simulink model "General_2_2025a"  (R2025a)
settings: Solver=ode45  StartTime=0.0  StopTime=inf  FixedStep=.1  RelTol=1e-3
undefined symbols (not defined in the file or in its folder): CR, dspblkCoreblockFVToolHelper, gcbh, LF, R_vec
libraries: instrumentseriallib x3, slpidlib x1, simulink x1
settings Model: Creator=aceve  LastModifiedBy=diego

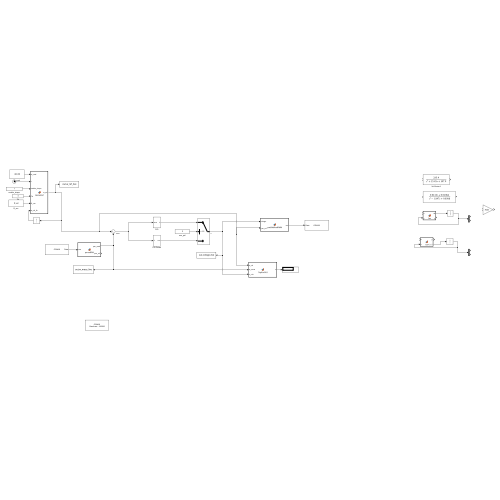
[thumbnail: Simulink's stored preview of the top-level diagram]
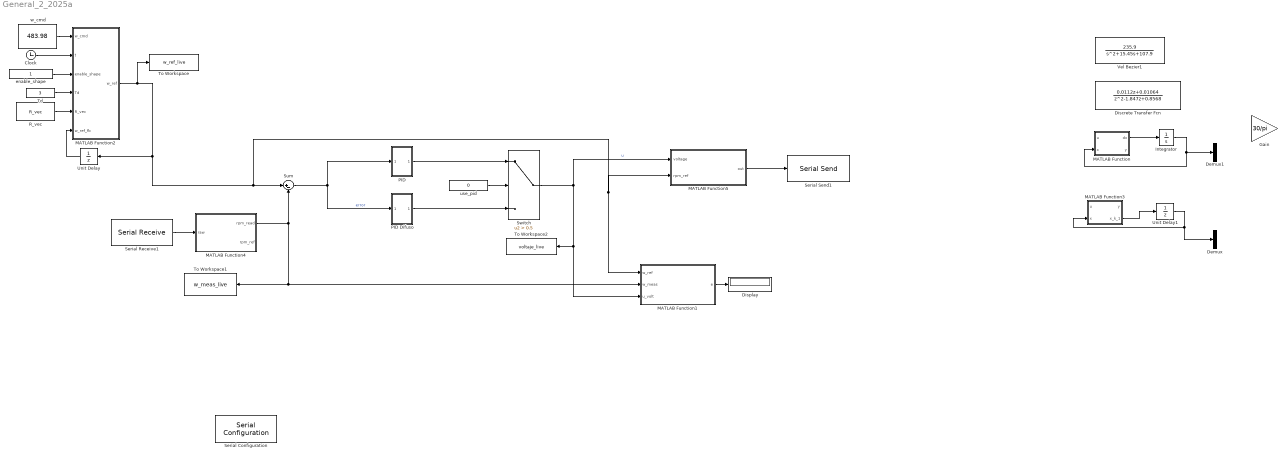
== system General_2_2025a ==
  Clock : Clock
  Demux : Demux  Outputs=2
  Demux1 : Demux  Outputs=2
  Discrete Transfer Fcn : DiscreteTransferFcn  LoadFcn=dspblkCoreblockFVToolHelper(gcbh,'load');  Numerator=[0.0112 0.01064 ]  Denominator=[1 -1.847 0.8568]
      settings: CopyFcn=dspblkCoreblockFVToolHelper(gcbh,'copy');  DeleteFcn=dspblkCoreblockFVToolHelper(gcbh,'close');  ModelCloseFcn=dspblkCoreblockFVToolHelper(gcbh,'close');  PreSaveFcn=dspblkCoreblockFVToolHelper(gcbh,'presave');  PostSaveFcn=dspblkCoreblockFVToolHelper(gcbh,'postsave');  CloseFcn=dspblkCoreblockFVToolHelper(gcbh,'close');
  Display : Display
  Gain : Gain  Gain=30/pi
  Integrator : Integrator  InitialCondition=[0;0]
  MATLAB Function : MATLAB Function  TreatAsAtomicUnit=on
  MATLAB Function1 : MATLAB Function  TreatAsAtomicUnit=on
  MATLAB Function2 : MATLAB Function  TreatAsAtomicUnit=on
  MATLAB Function3 : MATLAB Function  TreatAsAtomicUnit=on
  MATLAB Function4 : MATLAB Function  TreatAsAtomicUnit=on
  MATLAB Function5 : MATLAB Function  TreatAsAtomicUnit=on
  PID : Subsystem
  PID Difuso : Subsystem
  R_vec : Constant  Value=R_vec  SampleTime=-1
  Serial Configuration : instrumentseriallib/Serial Configuration  Priority=-200000  PortSel=COM19  Port=COM19  ComPort=COM19  BaudRate=115200  DataBits=8  Parity=none  StopBits=1  ByteOrder=little-endian  FlowControl=none  Timeout=10  SimulateUsing=Interpreted execution  BlockInModel=on  aMode=1
  Serial Receive1 : instrumentseriallib/Serial Receive  Priority=1  PortSel=COM19  Port=COM19  ComPort=COM19  DataType=int16  SaveDataType=uint8  ToggleHeader=off  Header=[]  ToggleDataSize=on  DataSize=[2 1]  ToggleTerminator=off  Terminator=CR/LF ('\r\n')  CustomTerminator=[]  InputFormat=Column major  EnableBlockingMode=on  ActionDataUnavailable=Output last received value  ActionWhenDataUnavailable=Output last received value  CustomValue=0  SampleTime=0.01  SimulateUsing=Interpreted execution  BlockInModel=on  aMode=1  LibraryInUse=instrumentlib
  Serial Send1 : instrumentseriallib/Serial Send  Priority=1  PortSel=COM19  Port=COM19  ComPort=COM19  Header=[]  Terminator=<none>  CustomTerminator=[]  EnableBlockingMode=off  SimulateUsing=Interpreted execution  BlockInModel=on  aMode=1
  Sum : Sum  Inputs=|+-
  Switch : Switch  Criteria=u2 > Threshold  Threshold=0.5  SaturateOnIntegerOverflow=off  InputSameDT=off
  Td : Constant  Value=3  SampleTime=-1
  To Workspace : ToWorkspace  VariableName=w_ref_live  SampleTime=-1
      settings: MaxDataPoints=1
  To Workspace1 : ToWorkspace  VariableName=w_meas_live  SampleTime=-1
      settings: MaxDataPoints=1
  To Workspace2 : ToWorkspace  VariableName=voltaje_live  SampleTime=-1
      settings: MaxDataPoints=1
  Unit Delay : UnitDelay  SampleTime=-1  HasFrameUpgradeWarning=on
  Unit Delay1 : UnitDelay  InitialCondition=[0;0]  SampleTime=-1  HasFrameUpgradeWarning=on
  Vel Bezier1 : TransferFcn  Numerator=[235.9]  Denominator=[1 15.45 107.9]
  enable_shape : Constant  SampleTime=-1
  use_pid : Constant  Value=0  SampleTime=-1
  w_cmd : Constant  Value=483.98  SampleTime=-1
  wires:
  PID/1(Out1) -> Switch/1
  use_pid/1 -> Switch/2
  Sum/1 -> PID/1(error), PID Difuso/1(In1)  "error"
  MATLAB Function2/1(w_ref) -> Sum/1, MATLAB Function1/1(w_ref), MATLAB Function5/2(rpm_ref), Unit Delay/1, To Workspace/1
  MATLAB Function1/1(e) -> Display/1
  R_vec/1 -> MATLAB Function2/5(R_vec)
  Clock/1 -> MATLAB Function2/2(t)
  Td/1 -> MATLAB Function2/4(Td)
  Unit Delay/1 -> MATLAB Function2/6(w_ref_fb)
  w_cmd/1 -> MATLAB Function2/1(w_cmd)
  enable_shape/1 -> MATLAB Function2/3(enable_shape)
  PID Difuso/1(out) -> Switch/3
  Switch/1 -> MATLAB Function1/3(u_volt), To Workspace2/1, MATLAB Function5/1(voltage)  "u"
  Integrator/1 -> Demux1/1, MATLAB Function/2(x)
  MATLAB Function/1(dx) -> Integrator/1
  MATLAB Function3/2(x_k_1) -> Unit Delay1/1
  Unit Delay1/1 -> Demux/1, MATLAB Function3/2(x)
  Serial Receive1/1 -> MATLAB Function4/1(raw)
  MATLAB Function5/1(out) -> Serial Send1/1
  MATLAB Function4/1(rpm_read) -> MATLAB Function1/2(w_meas), To Workspace1/1, Sum/2

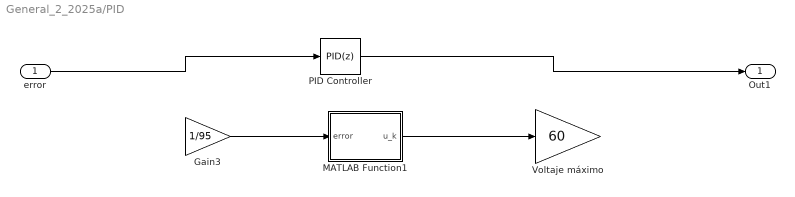
== system General_2_2025a/PID ==
  error : Inport
  Gain3 : Gain  Gain=1/95
  MATLAB Function1 : MATLAB Function  TreatAsAtomicUnit=on
  PID Controller : slpidlib/PID Controller  Controller=PID  Form=Parallel  TimeDomain=Discrete-time  UseExternalTs=off  SampleTime=0.01  IntegratorMethod=Forward Euler  FilterMethod=Forward Euler  ControllerParametersSource=internal  P=1.4156  I=177.0763  UseKiTs=off  D=0.038567  UseExternalDerivativeSource=off  N=9968.78766  UseFilter=on  TunerSelectOption=Transfer Function Based (PID Tuner App)  InitialConditionSource=internal  InitialConditionForIntegrator=0  InitialConditionForFilter=0  DifferentiatorICPrevScaledInput=0  ExternalReset=none  TrackingMode=off  Kt=1  LimitOutput=off  SatLimitsSource=internal  UpperSaturationLimit=inf  LowerSaturationLimit=-inf  LinearizeAsGain=on  AntiWindupMode=none  Kb=1  LimitIntegrator=off  UpperIntegratorSaturationLimit=inf  LowerIntegratorSaturationLimit=-inf  POutMin=[]  POutMax=[]  IOutMin=[]  IOutMax=[]  DOutMin=[]  DOutMax=[]  NOutMin=[]  NOutMax=[]  SumOutMin=[]  SumOutMax=[]  SaturationOutMin=[]  SaturationOutMax=[]  PParamMin=[]  PParamMax=[]  IParamMin=[]  IParamMax=[]  DParamMin=[]  DParamMax=[]  NParamMin=[]  NParamMax=[]  KbParamMin=[]  KbParamMax=[]  KtParamMin=[]  KtParamMax=[]  KbOutMin=[]  KbOutMax=[]  KtOutMin=[]  KtOutMax=[]  IntegratorOutMin=[]  IntegratorOutMax=[]  FilterOutMin=[]  FilterOutMax=[]  SumI1OutMin=[]  SumI1OutMax=[]  SumI2OutMin=[]  SumI2OutMax=[]  SumI3OutMin=[]  SumI3OutMax=[]  SumI4OutMin=[]  SumI4OutMax=[]  SumDOutMin=[]  SumDOutMax=[]  DifferentiatorOutMin=[]  DifferentiatorOutMax=[]  FilterDiffOutCoefMin=[]  FilterDiffOutCoefMax=[]  ReciprocalOutMin=[]  ReciprocalOutMax=[]  SumDenOutMin=[]  SumDenOutMax=[]  SumNumOutMin=[]  SumNumOutMax=[]  DivideOutMin=[]  DivideOutMax=[]  UdiffTsProdOutMin=[]  UdiffTsProdOutMax=[]  NTsProdOutMin=[]  NTsProdOutMax=[]  UintegralTsProdOutMin=[]  UintegralTsProdOutMax=[]  UngainTsProdOutMin=[]  UngainTsProdOutMax=[]  ClampingZeroOutDataTypeStr=Inherit: Inherit via back propagation  ClampingZeroOutMin=[]  ClampingZeroOutMax=[]  FilterDenConstantOutDataTypeStr=Inherit: Inherit via back propagation  FilterDenConstantOutMin=[]  FilterDenConstantOutMax=[]  PCopyOutDataTypeStr=Inherit: Inherit via back propagation  PCopyOutMin=[]  PCopyOutMax=[]  NCopyOutDataTypeStr=Inherit: Inherit via back propagation  NCopyOutMin=[]  NCopyOutMax=[]  IntegratorContinuousStateAttributes=''  IntegratorStateMustResolveToSignalObject=off  IntegratorRTWStateStorageClass=Auto  FilterContinuousStateAttributes=''  FilterStateMustResolveToSignalObject=off  FilterRTWStateStorageClass=Auto  ParallelPVariant=InternalParameters  IdealPVariant=Disabled  IVariant=InternalParameters  DVariant=InternalParameters  IntegratorVariant=Discrete  SatVariant=Disabled  AWVariant=Passthrough  PCopyVariant=Disabled  TRVariant=Disabled  FdbkBlocksVariant=Forward  IdealPFdbkVariant=Disabled  SatFdbkVariant=Disabled  DerivativeFilterVariant=ForwardEulerFilter  NVariant=InternalParameters  NCopyVariant=Disabled  FilterICVariant=InternalICsFilter  IntegratorICVariant=InternalICs  ExternalResetVariant=Disabled  TRSumVariant=Passthrough  SumFdbkVariant=Disabled  SumVariant=Sum_PID  TsampFilterVariant=InternalTs  TsampNgainVariant=Passthrough  TsampIntegralVariant=Disabled_SignalSpec  ExternalSaturationOutDataTypeStr=Inherit: Same as second input  DerivativeSourceVariant=ErrorSignal  PreIntVariant=InternalPreInt
  Voltaje máximo : Gain  Gain=60
  Out1 : Outport
  wires:
  Gain3/1 -> MATLAB Function1/1(error)
  MATLAB Function1/1(u_k) -> Voltaje máximo/1
  error/1 -> PID Controller/1
  PID Controller/1 -> Out1/1

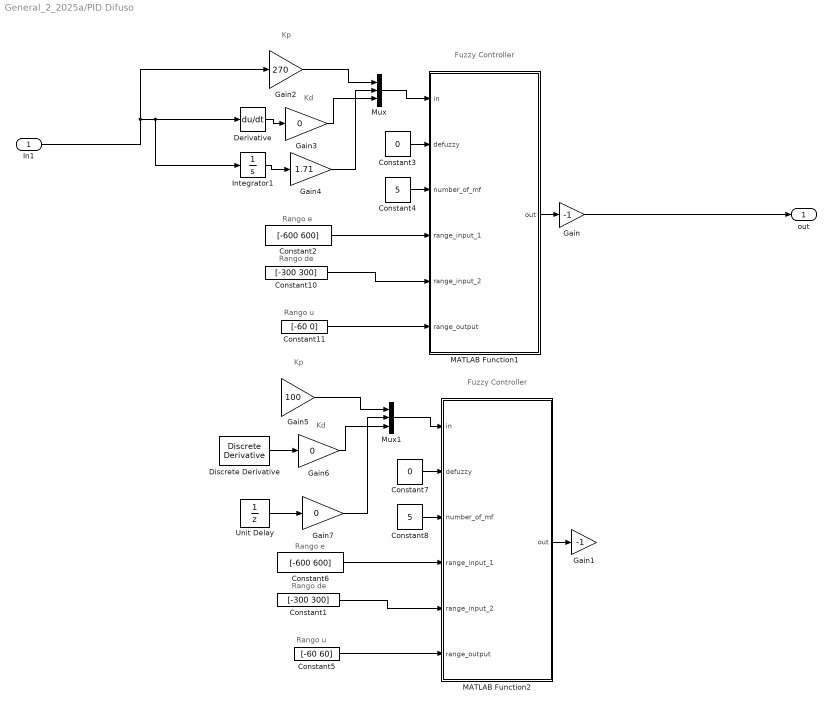
== system General_2_2025a/PID Difuso ==
  note: Rango e
  note: Kd
  note: Fuzzy Controller
  note: Kp
  note: Rango u
  note: Rango de
  note: Rango e
  note: Kd
  note: Fuzzy Controller
  note: Kp
  note: Rango u
  note: Rango de
  In1 : Inport
  Constant1 : Constant  Value=[-300 300]
  Constant10 : Constant  Value=[-300 300]
  Constant11 : Constant  Value=[-60 0]
  Constant2 : Constant  Value=[-600 600]
  Constant3 : Constant  Value=0
  Constant4 : Constant  Value=5
  Constant5 : Constant  Value=[-60 60]
  Constant6 : Constant  Value=[-600 600]
  Constant7 : Constant  Value=0
  Constant8 : Constant  Value=5
  Derivative : Derivative
  Discrete Derivative : simulink/Discrete/Discrete Derivative  gainval=1.0  ICPrevScaledInput=0.0  OutMin=[]  OutMax=[]  OutDataType=fixdt(1, 16)  OutScaling=2^-10  DoSatur=off
  Gain : Gain  Gain=-1
  Gain1 : Gain  Gain=-1
  Gain2 : Gain  Gain=270
  Gain3 : Gain  Gain=0
  Gain4 : Gain  Gain=1.71
  Gain5 : Gain  Gain=100
  Gain6 : Gain  Gain=0
  Gain7 : Gain  Gain=0
  Integrator1 : Integrator
  MATLAB Function1 : MATLAB Function  TreatAsAtomicUnit=on
  MATLAB Function2 : MATLAB Function  TreatAsAtomicUnit=on
  Mux : Mux  Inputs=3
  Mux1 : Mux  Inputs=3
  Unit Delay : UnitDelay  SampleTime=-1  HasFrameUpgradeWarning=on
  out : Outport
  wires:
  Constant4/1 -> MATLAB Function1/3(number_of_mf)
  Constant3/1 -> MATLAB Function1/2(defuzzy)
  Derivative/1 -> Gain3/1
  Mux/1 -> MATLAB Function1/1(in)
  Constant10/1 -> MATLAB Function1/5(range_input_2)
  Gain3/1 -> Mux/3
  Constant11/1 -> MATLAB Function1/6(range_output)
  Constant2/1 -> MATLAB Function1/4(range_input_1)
  Integrator1/1 -> Gain4/1
  Gain4/1 -> Mux/2
  Gain2/1 -> Mux/1
  MATLAB Function1/1(out) -> Gain/1
  MATLAB Function2/1(out) -> Gain1/1
  Gain5/1 -> Mux1/1
  Gain7/1 -> Mux1/2
  Unit Delay/1 -> Gain7/1
  Constant6/1 -> MATLAB Function2/4(range_input_1)
  Constant5/1 -> MATLAB Function2/6(range_output)
  Gain6/1 -> Mux1/3
  Constant1/1 -> MATLAB Function2/5(range_input_2)
  Mux1/1 -> MATLAB Function2/1(in)
  Discrete Derivative/1 -> Gain6/1
  Constant7/1 -> MATLAB Function2/2(defuzzy)
  Constant8/1 -> MATLAB Function2/3(number_of_mf)
  In1/1 -> Integrator1/1, Derivative/1, Gain2/1
  Gain/1 -> out/1

== matlab function General_2_2025a/MATLAB Function5 ==
  data: voltage input; rpm_ref input; out output
function out = packRefAndPWM(voltage, rpm_ref)
v_min = 0;
v_max = 30;

pwm_min = 0;
pwm_max = 65535;

% Escalado lineal
pwm_raw = (voltage - v_min) * (pwm_max - pwm_min) / (v_max - v_min) + pwm_min;

% Saturación
if pwm_raw > pwm_max * 0.9
    pwm_raw = pwm_max * 0.9;
elseif pwm_raw < pwm_max * 0.1
    pwm_raw = pwm_max * 0.1;
end

pwm_u16 = uint16(pwm_raw);
rpm_ref_u16 = uint16(rpm_ref);

out = uint16([rpm_ref_u16, pwm_u16]);
end

== matlab function General_2_2025a/PID Difuso/MATLAB Function1 ==
  data: in input; out output; defuzzy input; number_of_mf input; range_input_1 input; range_input_2 input; range_output input
function out = fcn(in, defuzzy, number_of_mf, range_input_1, range_input_2, range_output)
% CONTROLADOR FUZZY PID (Fuzzy PD + I)
% in: [error_scaled, d_error_scaled, integral_scaled]
% defuzzy: 0 = COG, 1 = CA
% range_input_1/2: [min, max] (Universo para PD)
% range_output: [min, max] (Universo para Salida Final, ej: [6, 54])

% === 1. Preparar divisiones ===
n = number_of_mf;
div1 = linspace(range_input_1(1), range_input_1(2), n); % error
div2 = linspace(range_input_2(1), range_input_2(2), n); % d_error

% El universo de salida del PD difuso. 
% Lo definimos igual que el rango de salida final por simplicidad.
div_out = linspace(range_output(1), range_output(2), n);

% === 2. Calcular membresías de entrada (solo para PD) ===
mu_e = compute_memberships(in(1), div1);
mu_de = compute_memberships(in(2), div2);

% === 3. Definir FAM (PD) ===
FAM = zeros(n, n);
middle_val = (n + 1) / 2;
middle_ij = middle_val*2;
for i = 1:n
    for j = 1:n
        v = middle_val + middle_ij - (i + j);
        if v > n, v = n; end
        if v < 1, v = 1; end
        FAM(i,j) = v;
    end
end

% === 4. Activaciones de reglas (PD) ===
rule_heights = zeros(n,n);
for i = 1:n
    for j = 1:n
        h = min(mu_e(i), mu_de(j));
        rule_heights(i,j) = h;
    end
end
% Max activación por salida
mu_out = zeros(1,n);
for k = 1:n
    % Encuentra todas las reglas (i,j) que tienen la salida k
    mask = (FAM == k);
    if any(mask(:)) % Evita max([]) si una etiqueta de salida no se usa
        mu_out(k) = max(rule_heights(mask));
    else
        mu_out(k) = 0;
    end
end

% === 5. Defuzzificación (Cálculo de la Salida PD) ===
% Usamos un valor central robusto por si den == 0
midL = floor((n+1)/2);
midR = ceil((n+1)/2);
center_val = 0.5*(div_out(midL) + div_out(midR));

fuzzy_pd_out = center_val; % Valor por defecto

if defuzzy == 0
    % --- COG (Centroide) ---
    num = 0; den = 0;
    if n > 1
        step = div_out(2)-div_out(1);
    else
        step = 0; % Evitar error si n=1
    end
    base = 2*step; % base total de cada triángulo
    for k = 1:n
        h = mu_out(k);
        if h > 0
            top_base = (1-h)*base;
            A = h*(base+top_base)/2; % área del trapecio
            num = num + A*div_out(k);
            den = den + A;
        end
    end
    if den > eps
        fuzzy_pd_out = num/den;
    end
else
    % --- CA (Promedio Ponderado) ---
    num = sum(mu_out .* div_out);
    den = sum(mu_out);
    if den > eps
        fuzzy_pd_out = num/den;
    end
end

% === 6. COMBINACIÓN PID (Fuzzy PD + I) ===
% Sumamos la salida difusa PD con la entrada Integral (in(3))
out_unclamped = fuzzy_pd_out + in(3);

% === 7. SATURACIÓN DE SALIDA ===
% Forzamos la salida final a estar dentro del rango [6, 54]
if out_unclamped < range_output(1)
    out = range_output(1); % Mínimo 6V
elseif out_unclamped > range_output(2)
    out = range_output(2); % Máximo 54V
else
    out = out_unclamped;
end

end

% === Función Auxiliar de Membresías ===
function mu = compute_memberships(x, div)
n = length(div);
mu = zeros(1,n);
if x <= div(1)
    mu(1) = 1; return
elseif x >= div(end)
    mu(end) = 1; return
end
for i = 1:n-1
    x1 = div(i); x2 = div(i+1);
    den = x2 - x1;
    if den == 0, den = eps; end % Evitar división por cero
    
    if x >= x1 && x <= x2
        mu(i) = (x2 - x)/den;
        mu(i+1) = (x - x1)/den;
        return
    end
end
end

== matlab function General_2_2025a/MATLAB Function3 ==
  data: y output; x_k_1 output; u input; x input
function [y,x_k_1] = fcn(u, x)

x1 = x(1);
x2 = x(2);

x1_k_1_ =  1.847*x1 -0.8568*x2 + .125*u;
x2_k_1 = x1;

x_k_1 = [x1_k_1_;x2_k_1];
y = 0.0896*x1 + 0.0851*x2;

== matlab function General_2_2025a/MATLAB Function ==
  data: dx output; u input; y output; x input
function [dx, y] = fcn(u, x)
%#codegen
% Modelo DC motor (2 estados): x = [omega; i]
%   J*dω/dt = -b*ω + Kt*i
%   L*di/dt = -Kb*ω - R*i + u
% y = ω

% ---- parámetros (double explícito) ----
R  = 6.6;
L  = 8.15e-3;
Kb = 0.436;
Kt = 0.436;          % (tq. constante; igual a Kb si SI)
J  = 4.0e-3;
b  = 1.32e-3;

% ---- asegurar tamaños ----
x1 = x(1);           % ω
x2 = x(2);           % i

dx         = zeros(2,1);   % <- tamaño fijo para Simulink/Codegen
dx(1,1)    = -(b/J)*x1 + (Kt/J)*x2;
dx(2,1)    = -(Kb/L)*x1 - (R/L)*x2 + (1/L)*u;

y = x1;              % salida = velocidad
end

== matlab function General_2_2025a/MATLAB Function2 ==
  settings: updateMethod=DISCRETE
  data: w_cmd input; t input; w_ref output; enable_shape input; Td input; R_vec input; w_ref_fb input
function w_ref = BezierRef(w_cmd, t, enable_shape, Td, R_vec, w_ref_fb)
% =================================================================
% VERSIÓN 5 (Coeficientes R_vec y bug de comparación corregidos)
% =================================================================
%
% Entradas:
%   w_cmd     : setpoint deseado (de la GUI)
%   t         : tiempo absoluto (Clock)
%   enable_shape : 1 = perfilar, 0 = paso directo
%   Td        : duración de la transición [s]
%   R_vec     : [r1..r6] coeficientes del polinomio
%   w_ref_fb  : w_ref anterior (feedback vía Memory/Unit Delay)
%
% Salida:
%   w_ref     : referencia suavizada

% --- estados persistentes ---
persistent w0 wf t0 last_cmd is_initialized

% --- Lógica de inicialización en el primer paso de ejecución ---
if isempty(is_initialized) || t == 0 % Se reinicia si el tiempo es 0
    is_initialized = true; 
    
    w0 = w_ref_fb; 
    wf = w_cmd;
    t0 = t;
    last_cmd = w_cmd;
end

% --- FIX 1: Detecta cambio de comando con tolerancia ---
if abs(w_cmd - last_cmd) > 1e-6
    % Nuevo tramo desde el valor de salida actual (feedback) hacia w_cmd
    w0 = w_ref_fb;
    wf = w_cmd;
    t0 = t;
    last_cmd = w_cmd;
end

% Paso directo si está desactivado
if enable_shape == 0 || Td <= 0
    w_ref = w_cmd;
    % Asegurarse de que el estado interno se actualice para el próximo arranque
    w0 = w_cmd; 
    wf = w_cmd;
    last_cmd = w_cmd;
    return
end

% Progreso normalizado en [0,1]
s = (t - t0) / Td;

if s <= 0
    alpha = 0;
elseif s >= 1
    alpha = 1;
else
    % Bezier polinómico
    if numel(R_vec) < 6
        alpha = s; % Fallback a rampa lineal
    else
        % --- FIX 2: Validar que R_vec sea correcto ---
        % La suma de coeficientes alternados debe ser 1 para que alpha(1)=1.
        % (r1 - r2 + r3 - r4 + r5 - r6) == 1
        % Si no, se usa una rampa simple s^5.
        
        r1 = R_vec(1); r2 = R_vec(2); r3 = R_vec(3);
        r4 = R_vec(4); r5 = R_vec(5); r6 = R_vec(6);
        
        % Comprobamos si el vector R_vec está mal (la suma es != 1)
        if abs((r1 - r2 + r3 - r4 + r5 - r6) - 1.0) > 1e-3
            % Vector R_vec incorrecto. Usar rampa s^5 simple.
            alpha = s^5;
        else
            % Vector R_vec es válido, usar la fórmula completa
            alpha = (s.^5).*(r1 - r2*s + r3*s.^2 - r4*s.^3 + r5*s.^4 - r6*s.^5);
        end
    end
    
    % Clampeo por seguridad numérica
    if alpha < 0, alpha = 0; end
    if alpha > 1, alpha = 1; end
end

% Interpolación entre w0 y wf
w_ref = w0 + alpha*(wf - w0);

== matlab function General_2_2025a/PID/MATLAB Function1 ==
  settings: updateMethod=DISCRETE
  data: error input; u_k output
function u_k = PID(error)

% Esta función implementa el controlador PID discreto del código de Arduino.

% ENTRADA:

% error: El error actual e(k) = (referencia - medida)

% SALIDA:

% u_k: La señal de control saturada (entre 0.0 y 1.0)

% ===== Parámetros del Controlador (iguales a los de Arduino) =====

Kc = 0.15;

Ti = 0.05;

Td = 0.00;

N = 100;

Ts_s = 0.01; % Periodo de muestreo en segundos (10 ms)

% ===== Variables de Estado (persisten entre llamadas) =====

% Se declaran como 'persistent' para que guarden su valor,

% igual que las variables globales en Arduino.

persistent error_prev integral_prev derivative_prev

% ===== Inicialización en la primera ejecución =====

% La primera vez que se llama a la función, las variables están vacías.

if isempty(error_prev)

error_prev = 0.0;

integral_prev = 0.0;

derivative_prev = 0.0;

end

% ================================================================

% ===== LÓGICA DE CONTROL PID (Traducción directa de C++) ========

% ================================================================

% 2. Calcular término Proporcional: p(k) = Kc * e(k)

p_k = Kc * error;

% 3. Calcular término Integral: i(k) = i(k-1) + (h*Kc/Ti) * e(k)

i_k = integral_prev + (Kc * Ts_s / Ti) * error;

% 4. Calcular término Derivativo: d(k) = c1*d(k-1) + c2*e(k) - c2*e(k-1)

c1 = 1.0 / (1.0 + Ts_s * N);

c2 = (Kc * Td * N) / (1.0 + Ts_s * N);

d_k = c1 * derivative_prev + c2 * (error - error_prev);

% 5. Calcular la salida de control total: u(k) = p(k) + i(k) + d(k)

u_k_total = p_k + i_k + d_k;

% --- Saturación y Anti-Windup ---

u_k_saturado = u_k_total;

if u_k_saturado > 1.0

u_k_saturado = 1.0;

end

if u_k_saturado < 0.0

u_k_saturado = 0.0;

end

% --- Actualización de estados para la siguiente iteración ---

% Anti-Windup: Actualizar el término integral solo si no hay saturación

if u_k_total == u_k_saturado

integral_prev = i_k;

end

derivative_prev = d_k;

error_prev = error;

% Asignar la salida final de la función

u_k = u_k_saturado;

end

== matlab function General_2_2025a/MATLAB Function4 ==
  data: raw input; rpm_read output; rpm_ref output
function [rpm_read, rpm_ref] = parseRPM(raw)
%#codegen
% raw: 1x2 uint16 vector received from ESP32
% rpm_read: measured RPM from encoder
% rpm_ref:  reference RPM echoed back from ESP32

rpm_read = double(raw(1));   % first  uint16 from ESP32
rpm_ref  = double(raw(2));   % second uint16 from ESP32
end

== matlab function General_2_2025a/MATLAB Function1 ==
  data: w_ref input; e output; w_meas input; u_volt input
function e = TapForGUI(w_ref, w_meas, u_volt)
% Publica las señales para la GUI y devuelve el error.
% Entradas:
%   w_ref  - velocidad deseada
%   w_meas - velocidad medida
%   u_volt - voltaje (señal de control 'u')
%
% Salida:
%   e      - error (w_ref - w_meas)

assignin('base','w_ref_live',w_ref);
assignin('base','w_meas_live',w_meas);
assignin('base','voltaje_live',u_volt); % <-- LÍNEA AÑADIDA
assignin('base','err_live',w_ref - w_meas);

e = w_ref - w_meas;

== matlab function General_2_2025a/PID Difuso/MATLAB Function2 ==
  data: in input; out output; defuzzy input; number_of_mf input; range_input_1 input; range_input_2 input; range_output input
function out = fcn(in, defuzzy, number_of_mf, range_input_1, range_input_2, range_output)
% CONTROLADOR FUZZY PID (Fuzzy PD + I)
% in: [error_scaled, d_error_scaled, integral_scaled]
% defuzzy: 0 = COG, 1 = CA
% range_input_1/2: [min, max] (Universo para PD)
% range_output: [min, max] (Universo para Salida Final, ej: [6, 54])

% === 1. Preparar divisiones ===
n = number_of_mf;
div1 = linspace(range_input_1(1), range_input_1(2), n); % error
div2 = linspace(range_input_2(1), range_input_2(2), n); % d_error

% El universo de salida del PD difuso. 
% Lo definimos igual que el rango de salida final por simplicidad.
div_out = linspace(range_output(1), range_output(2), n);

% === 2. Calcular membresías de entrada (solo para PD) ===
mu_e = compute_memberships(in(1), div1);
mu_de = compute_memberships(in(2), div2);

% === 3. Definir FAM (PD) ===
FAM = zeros(n, n);
middle_val = (n + 1) / 2;
middle_ij = middle_val*2;
for i = 1:n
    for j = 1:n
        v = middle_val + middle_ij - (i + j);
        if v > n, v = n; end
        if v < 1, v = 1; end
        FAM(i,j) = v;
    end
end

% === 4. Activaciones de reglas (PD) ===
rule_heights = zeros(n,n);
for i = 1:n
    for j = 1:n
        h = min(mu_e(i), mu_de(j));
        rule_heights(i,j) = h;
    end
end
% Max activación por salida
mu_out = zeros(1,n);
for k = 1:n
    % Encuentra todas las reglas (i,j) que tienen la salida k
    mask = (FAM == k);
    if any(mask(:)) % Evita max([]) si una etiqueta de salida no se usa
        mu_out(k) = max(rule_heights(mask));
    else
        mu_out(k) = 0;
    end
end

% === 5. Defuzzificación (Cálculo de la Salida PD) ===
% Usamos un valor central robusto por si den == 0
midL = floor((n+1)/2);
midR = ceil((n+1)/2);
center_val = 0.5*(div_out(midL) + div_out(midR));

fuzzy_pd_out = center_val; % Valor por defecto

if defuzzy == 0
    % --- COG (Centroide) ---
    num = 0; den = 0;
    if n > 1
        step = div_out(2)-div_out(1);
    else
        step = 0; % Evitar error si n=1
    end
    base = 2*step; % base total de cada triángulo
    for k = 1:n
        h = mu_out(k);
        if h > 0
            top_base = (1-h)*base;
            A = h*(base+top_base)/2; % área del trapecio
            num = num + A*div_out(k);
            den = den + A;
        end
    end
    if den > eps
        fuzzy_pd_out = num/den;
    end
else
    % --- CA (Promedio Ponderado) ---
    num = sum(mu_out .* div_out);
    den = sum(mu_out);
    if den > eps
        fuzzy_pd_out = num/den;
    end
end

% === 6. COMBINACIÓN PID (Fuzzy PD + I) ===
% Sumamos la salida difusa PD con la entrada Integral (in(3))
out_unclamped = fuzzy_pd_out + in(3);

% === 7. SATURACIÓN DE SALIDA ===
% Forzamos la salida final a estar dentro del rango [6, 54]
if out_unclamped < range_output(1)
    out = range_output(1); % Mínimo 6V
elseif out_unclamped > range_output(2)
    out = range_output(2); % Máximo 54V
else
    out = out_unclamped;
end

end

% === Función Auxiliar de Membresías ===
function mu = compute_memberships(x, div)
n = length(div);
mu = zeros(1,n);
if x <= div(1)
    mu(1) = 1; return
elseif x >= div(end)
    mu(end) = 1; return
end
for i = 1:n-1
    x1 = div(i); x2 = div(i+1);
    den = x2 - x1;
    if den == 0, den = eps; end % Evitar división por cero
    
    if x >= x1 && x <= x2
        mu(i) = (x2 - x)/den;
        mu(i+1) = (x - x1)/den;
        return
    end
end
end
